simulink model "GFLIB_Lut1D_BAM"  (Simulink 7.3)
settings: Solver=ode45  StartTime=0.0  StopTime=10.0  RelTol=1e-3
undefined symbols (not defined in the file): pf32Table, s32MidIdx, u32ShamOffset
settings Model: Creator=B17364  LastModifiedBy=B17364

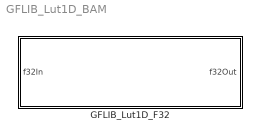
== system GFLIB_Lut1D_BAM ==
  GFLIB_Lut1D_F32 : Subsystem  mask(GFLIB_Lut1D_F32){u32ShamOffset=u32ShamOffset, pf32Table=pf32Table, s32MidIdx=s32MidIdx}
      mask help: Bit accurate model of Lut1D function.
      mask init:
      | pos = get_param(gcb, 'Position');width = pos(3) - pos(1); height = pos(4) - pos(2);tX=width/2;tY=height*0.9;
      mask Display: color('black');port_label('input',1,'f32In');port_label('output',1,'f32Out');color('black');disp('GFLIB_Lut1D_F32');color('blue');text(tX,tY, 'BAM', 'horizontalAlignment', 'center');

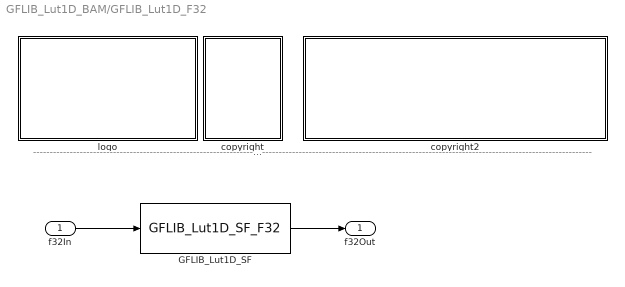
== system GFLIB_Lut1D_BAM/GFLIB_Lut1D_F32 ==
  note: ---------------------------------------------------------------------------------------------------------------------------------------------------------------------------------------------------
  f32In : Inport  OutDataType=fixdt(1, 16)  OutScaling=2^0
  GFLIB_Lut1D_SF : S-Function  FunctionName=GFLIB_Lut1D_SF_F32  Parameters=u32ShamOffset,pf32Table,s32MidIdx  EnableBusSupport=off
  copyright : Subsystem
      mask Display: text(10,90,'FILE:');text(10,75,'DESRIPTION:')text(10,60,'COPYRIGHT:')text(10,45,'VERSION:')text(10,30,'DATE:')
  copyright2 : Subsystem
      mask Display: text(10,90,'GFLIB_Lut1D_BAM_F32.mdl');text(10,75,'One dimensional Look-up table function');text(10,60,'Freescale')text(10,45,'0.1');text(10,30,'17-Jun-2013');
  logo : Subsystem
      mask Display: image(imread('logo.jpg'))
  f32Out : Outport  OutDataType=fixdt(1, 16)  OutScaling=2^0
  wires:
  f32In/1 -> GFLIB_Lut1D_SF/1
  GFLIB_Lut1D_SF/1 -> f32Out/1

== system GFLIB_Lut1D_BAM/GFLIB_Lut1D_F32/copyright ==

== system GFLIB_Lut1D_BAM/GFLIB_Lut1D_F32/copyright2 ==

== system GFLIB_Lut1D_BAM/GFLIB_Lut1D_F32/logo ==
